simulink model "copter_simulink_control_trajectory_circle4"  (R2018b)
settings: Solver=ode45  StartTime=0.0  StopTime=200  FixedStep=.001  MaxStep=.05  MinStep=0.0001  RelTol=1e-3  EnableMultiTasking=on
libraries: simulink x10
settings Model: Creator=bengiami  LastModifiedBy=bengiami
settings SolverCC: MaxConsecutiveZCs=100  AutoInsertRateTranBlk=on
settings DataIOCC: LimitDataPoints=on  SaveFormat=Array  SaveOutput=off  SaveTime=off
settings OptimizationCC: DefaultParameterBehavior=Inlined  InlineInvariantSignals=on  StateBitsets=on  DataBitsets=on  ZeroExternalMemoryAtStartup=off  ZeroInternalMemoryAtStartup=off  NoFixptDivByZeroProtection=on  LifeSpan=1
settings DebuggingCC: AlgebraicLoopMsg=none  MaxConsecutiveZCsMsg=none  SolverPrmCheckMsg=warning  SFUnexpectedBacktrackingDiag=warning  SFNoUnconditionalDefaultTransitionDiag=warning  SFExecutionAtInitializationDiag=none
settings HardwareCC: ProdBitPerPointer=32  ProdBitPerSizeT=32  ProdBitPerPtrDiffT=32  ProdLargestAtomicFloat=None  ProdIntDivRoundTo=Floor  ProdWordSize=32  ProdHWDeviceType=Generic->Custom
settings ModelReferenceCC: PropagateSignalLabelsOutOfModel=off
settings SFSimCC: SimUseLocalCustomCode=off  MATLABDynamicMemAlloc=off
settings RTWCC: SystemTargetFile=ert.tlc  TLCOptions=-p0  GenCodeOnly=on  TemplateMakefile=ert_default_tmf  GenerateReport=on  RTWVerbose=off  RTWUseLocalCustomCode=off  IncludeHyperlinkInReport=on  LaunchReport=on
settings CodeAppCC: ForceParamTrailComments=on  IgnoreCustomStorageClasses=off  SimulinkDataObjDesc=on  CustomSymbolStrGlobalVar=rt$N$M  CustomSymbolStrType=$N$M  CustomSymbolStrFcn=$N$M$F  CustomSymbolStrMacro=$N$M  InsertBlockDesc=on  StateflowObjectComments=on
settings ERTTargetCC: CodeReplacementLibrary=ISO_C  MultiwordLength=2048  GenerateSampleERTMain=on  IncludeMdlTerminateFcn=off  SuppressErrorStatus=on  SupportAbsoluteTime=off  PurelyIntegerCode=on  SupportNonFinite=off  SupportComplex=off  InlinedParameterPlacement=NonHierarchical  RootIOFormat=Structure reference  ERTCustomFileTemplate=example_file_process.tlc  ConvertIfToSwitch=off  SuppressUnreachableDefaultCases=off
settings ConfigComp: CovMetricSettings=dw  CovHtmlReporting=on  CovSaveCumulativeToWorkspaceVar=on  CovSaveSingleToWorkspaceVar=on  CovExternalEMLEnable=off  CovSFcnEnable=off

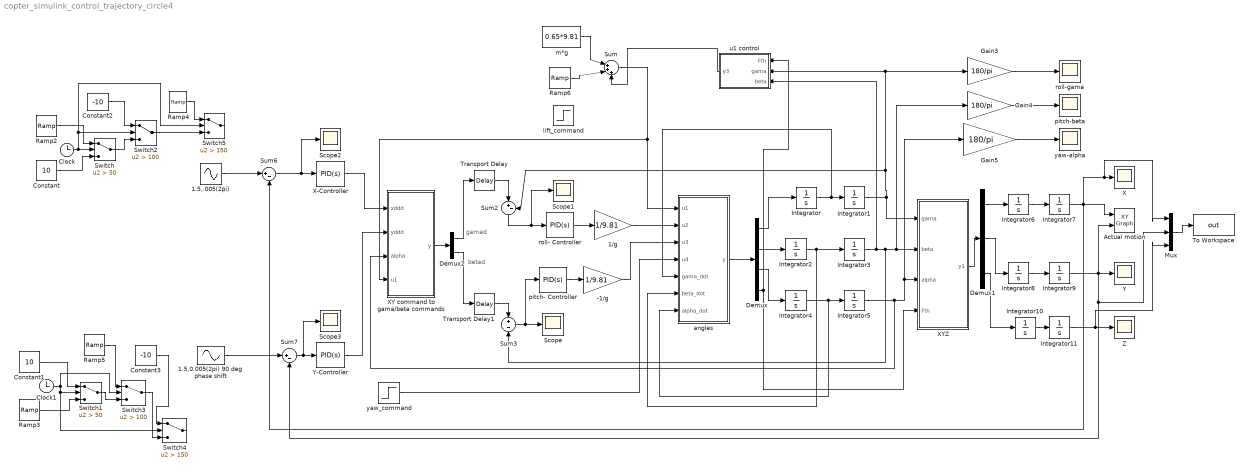
== system copter_simulink_control_trajectory_circle4 ==
  note: betad
  note: gamad
  -1/g : Gain  Gain=1/9.81
  1.5,.005(2pi) : Sin  Amplitude=10  Frequency=0.005*(2*pi)  SampleTime=0
  1.5,0.005(2pi) 90 deg phase shift : Sin  Amplitude=10  Frequency=0.005*(2*pi)  Phase=pi/2  SampleTime=0
  1/g : Gain  Gain=1/9.81
  Actual motion : simulink/Sinks/XY Graph  xmin=-25  xmax=25  ymin=-25  ymax=25  st=-1
  Clock : Clock
  Clock1 : Clock
  Constant : Constant  Value=10
  Constant1 : Constant  Value=10
  Constant2 : Constant  Value=-10
  Constant3 : Constant  Value=-10
  Demux : Demux
  Demux1 : Demux  Outputs=3
  Demux2 : Demux  Outputs=2
  Gain3 : Gain  Gain=180/pi
  Gain4 : Gain  Gain=180/pi
  Gain5 : Gain  Gain=180/pi
  Integrator{,1..8,10..11} (11 alike) : Integrator
  Integrator9 : Integrator  InitialCondition=10
  Mux : Mux  Inputs=3
  Ramp2 : simulink/Sources/Ramp  slope=-0.4  start=50  InitialOutput=10
  Ramp3 : simulink/Sources/Ramp  slope=0.4  start=0  InitialOutput=-10
  Ramp4 : simulink/Sources/Ramp  slope=0.4  start=150  InitialOutput=-10
  Ramp5 : simulink/Sources/Ramp  slope=-0.4  start=100  InitialOutput=10
  Ramp6 : simulink/Sources/Ramp  slope=-0.0000001  start=0  InitialOutput=0
  Scope{,1..3} (4 alike) : Scope
  Sum : Sum  Inputs=|+++
  Sum2 : Sum  Inputs=|+-
  Sum3 : Sum  Inputs=+-
  Sum6 : Sum  Inputs=|+-
  Sum7 : Sum  Inputs=|+-
  Switch : Switch  Criteria=u2 > Threshold  Threshold=50
  Switch1 : Switch  Criteria=u2 > Threshold  Threshold=50
  Switch2 : Switch  Criteria=u2 > Threshold  Threshold=100
  Switch3 : Switch  Criteria=u2 > Threshold  Threshold=100
  Switch4 : Switch  Criteria=u2 > Threshold  Threshold=150
  Switch5 : Switch  Criteria=u2 > Threshold  Threshold=150
  To Workspace : ToWorkspace  VariableName=out  SaveFormat=Timeseries  SampleTime=-1
  Transport Delay : TransportDelay  DelayTime=0.0001
  Transport Delay1 : TransportDelay  DelayTime=0.0001
  X : Scope
  X-Controller : simulink/Continuous/PID Controller  Controller=PID  Form=Parallel  TimeDomain=Continuous-time  SampleTime=1  IntegratorMethod=Forward Euler  FilterMethod=Forward Euler  ControllerParametersSource=internal  P=2  I=0.05  D=0.1  UseFilter=on  N=1000  TunerSelectOption=Transfer Function Based (PID Tuner App)  InitialConditionSource=internal  InitialConditionForIntegrator=0  InitialConditionForFilter=0  DifferentiatorICPrevScaledInput=0  ExternalReset=none  TrackingMode=off  Kt=1  LimitOutput=off  UpperSaturationLimit=inf  LowerSaturationLimit=-inf  LinearizeAsGain=on  AntiWindupMode=none  Kb=1  POutMin=[]  POutMax=[]  IOutMin=[]  IOutMax=[]  DOutMin=[]  DOutMax=[]  NOutMin=[]  NOutMax=[]  SumOutMin=[]  SumOutMax=[]  SaturationOutMin=[]  SaturationOutMax=[]  PParamMin=[]  PParamMax=[]  IParamMin=[]  IParamMax=[]  DParamMin=[]  DParamMax=[]  NParamMin=[]  NParamMax=[]  KbParamMin=[]  KbParamMax=[]  KtParamMin=[]  KtParamMax=[]  KbOutMin=[]  KbOutMax=[]  KtOutMin=[]  KtOutMax=[]  IntegratorOutMin=[]  IntegratorOutMax=[]  FilterOutMin=[]  FilterOutMax=[]  SumI1OutMin=[]  SumI1OutMax=[]  SumI2OutMin=[]  SumI2OutMax=[]  SumI3OutMin=[]  SumI3OutMax=[]  SumI4OutMin=[]  SumI4OutMax=[]  SumDOutMin=[]  SumDOutMax=[]  DifferentiatorOutMin=[]  DifferentiatorOutMax=[]  FilterDiffOutCoefMin=[]  FilterDiffOutCoefMax=[]  ReciprocalOutMin=[]  ReciprocalOutMax=[]  SumDenOutMin=[]  SumDenOutMax=[]  SumNumOutMin=[]  SumNumOutMax=[]  DivideOutMin=[]  DivideOutMax=[]  IntegratorContinuousStateAttributes=''  IntegratorStateMustResolveToSignalObject=off  IntegratorRTWStateStorageClass=Auto  FilterContinuousStateAttributes=''  FilterStateMustResolveToSignalObject=off  FilterRTWStateStorageClass=Auto  ParallelPVariant=InternalParameters  IdealPVariant=Disabled  IVariant=InternalParameters  DVariant=InternalParameters  IntegratorVariant=Continuous  SatVariant=Disabled  AWVariant=Passthrough  PCopyVariant=Disabled  TRVariant=Disabled  FdbkBlocksVariant=Forward  IdealPFdbkVariant=Disabled  SatFdbkVariant=Disabled  DerivativeFilterVariant=ContFilter  NVariant=InternalParameters  NCopyVariant=Disabled  FilterICVariant=InternalICsFilter  IntegratorICVariant=InternalICs  ExternalResetVariant=Disabled  TRSumVariant=Passthrough  SumFdbkVariant=Disabled  SumVariant=Sum_PID
  XY command to gama/beta commands : MATLAB Function  TreatAsAtomicUnit=on
  XYZ : MATLAB Function  TreatAsAtomicUnit=on
  Y : Scope
  Y-Controller : simulink/Continuous/PID Controller  Controller=PID  Form=Parallel  TimeDomain=Continuous-time  SampleTime=1  IntegratorMethod=Forward Euler  FilterMethod=Forward Euler  ControllerParametersSource=internal  P=2  I=0.05  D=0.13  UseFilter=on  N=1000  TunerSelectOption=Transfer Function Based (PID Tuner App)  InitialConditionSource=internal  InitialConditionForIntegrator=0  InitialConditionForFilter=0  DifferentiatorICPrevScaledInput=0  ExternalReset=none  TrackingMode=off  Kt=1  LimitOutput=off  UpperSaturationLimit=inf  LowerSaturationLimit=-inf  LinearizeAsGain=on  AntiWindupMode=none  Kb=1  POutMin=[]  POutMax=[]  IOutMin=[]  IOutMax=[]  DOutMin=[]  DOutMax=[]  NOutMin=[]  NOutMax=[]  SumOutMin=[]  SumOutMax=[]  SaturationOutMin=[]  SaturationOutMax=[]  PParamMin=[]  PParamMax=[]  IParamMin=[]  IParamMax=[]  DParamMin=[]  DParamMax=[]  NParamMin=[]  NParamMax=[]  KbParamMin=[]  KbParamMax=[]  KtParamMin=[]  KtParamMax=[]  KbOutMin=[]  KbOutMax=[]  KtOutMin=[]  KtOutMax=[]  IntegratorOutMin=[]  IntegratorOutMax=[]  FilterOutMin=[]  FilterOutMax=[]  SumI1OutMin=[]  SumI1OutMax=[]  SumI2OutMin=[]  SumI2OutMax=[]  SumI3OutMin=[]  SumI3OutMax=[]  SumI4OutMin=[]  SumI4OutMax=[]  SumDOutMin=[]  SumDOutMax=[]  DifferentiatorOutMin=[]  DifferentiatorOutMax=[]  FilterDiffOutCoefMin=[]  FilterDiffOutCoefMax=[]  ReciprocalOutMin=[]  ReciprocalOutMax=[]  SumDenOutMin=[]  SumDenOutMax=[]  SumNumOutMin=[]  SumNumOutMax=[]  DivideOutMin=[]  DivideOutMax=[]  IntegratorContinuousStateAttributes=''  IntegratorStateMustResolveToSignalObject=off  IntegratorRTWStateStorageClass=Auto  FilterContinuousStateAttributes=''  FilterStateMustResolveToSignalObject=off  FilterRTWStateStorageClass=Auto  ParallelPVariant=InternalParameters  IdealPVariant=Disabled  IVariant=InternalParameters  DVariant=InternalParameters  IntegratorVariant=Continuous  SatVariant=Disabled  AWVariant=Passthrough  PCopyVariant=Disabled  TRVariant=Disabled  FdbkBlocksVariant=Forward  IdealPFdbkVariant=Disabled  SatFdbkVariant=Disabled  DerivativeFilterVariant=ContFilter  NVariant=InternalParameters  NCopyVariant=Disabled  FilterICVariant=InternalICsFilter  IntegratorICVariant=InternalICs  ExternalResetVariant=Disabled  TRSumVariant=Passthrough  SumFdbkVariant=Disabled  SumVariant=Sum_PID
  Z : Scope
  angles : MATLAB Function  TreatAsAtomicUnit=on
  lift_command : Step  Time=0  After=0  SampleTime=0
  m*g : Constant  Value=0.65*9.81
  pitch- Controller : simulink/Continuous/PID Controller  Controller=PID  Form=Parallel  TimeDomain=Continuous-time  SampleTime=1  IntegratorMethod=Forward Euler  FilterMethod=Forward Euler  ControllerParametersSource=internal  P=4  I=0.05  D=0.1  UseFilter=on  N=1000  TunerSelectOption=Transfer Function Based (PID Tuner App)  InitialConditionSource=internal  InitialConditionForIntegrator=0  InitialConditionForFilter=0  DifferentiatorICPrevScaledInput=0  ExternalReset=none  TrackingMode=off  Kt=1  LimitOutput=off  UpperSaturationLimit=inf  LowerSaturationLimit=-inf  LinearizeAsGain=on  AntiWindupMode=none  Kb=1  POutMin=[]  POutMax=[]  IOutMin=[]  IOutMax=[]  DOutMin=[]  DOutMax=[]  NOutMin=[]  NOutMax=[]  SumOutMin=[]  SumOutMax=[]  SaturationOutMin=[]  SaturationOutMax=[]  PParamMin=[]  PParamMax=[]  IParamMin=[]  IParamMax=[]  DParamMin=[]  DParamMax=[]  NParamMin=[]  NParamMax=[]  KbParamMin=[]  KbParamMax=[]  KtParamMin=[]  KtParamMax=[]  KbOutMin=[]  KbOutMax=[]  KtOutMin=[]  KtOutMax=[]  IntegratorOutMin=[]  IntegratorOutMax=[]  FilterOutMin=[]  FilterOutMax=[]  SumI1OutMin=[]  SumI1OutMax=[]  SumI2OutMin=[]  SumI2OutMax=[]  SumI3OutMin=[]  SumI3OutMax=[]  SumI4OutMin=[]  SumI4OutMax=[]  SumDOutMin=[]  SumDOutMax=[]  DifferentiatorOutMin=[]  DifferentiatorOutMax=[]  FilterDiffOutCoefMin=[]  FilterDiffOutCoefMax=[]  ReciprocalOutMin=[]  ReciprocalOutMax=[]  SumDenOutMin=[]  SumDenOutMax=[]  SumNumOutMin=[]  SumNumOutMax=[]  DivideOutMin=[]  DivideOutMax=[]  IntegratorContinuousStateAttributes=''  IntegratorStateMustResolveToSignalObject=off  IntegratorRTWStateStorageClass=Auto  FilterContinuousStateAttributes=''  FilterStateMustResolveToSignalObject=off  FilterRTWStateStorageClass=Auto  ParallelPVariant=InternalParameters  IdealPVariant=Disabled  IVariant=InternalParameters  DVariant=InternalParameters  IntegratorVariant=Continuous  SatVariant=Disabled  AWVariant=Passthrough  PCopyVariant=Disabled  TRVariant=Disabled  FdbkBlocksVariant=Forward  IdealPFdbkVariant=Disabled  SatFdbkVariant=Disabled  DerivativeFilterVariant=ContFilter  NVariant=InternalParameters  NCopyVariant=Disabled  FilterICVariant=InternalICsFilter  IntegratorICVariant=InternalICs  ExternalResetVariant=Disabled  TRSumVariant=Passthrough  SumFdbkVariant=Disabled  SumVariant=Sum_PID
  pitch-beta : Scope
  roll- Controller : simulink/Continuous/PID Controller  Controller=PID  Form=Parallel  TimeDomain=Continuous-time  SampleTime=1  IntegratorMethod=Forward Euler  FilterMethod=Forward Euler  ControllerParametersSource=internal  P=4  I=0.05  D=0.1  UseFilter=on  N=1000  TunerSelectOption=Transfer Function Based (PID Tuner App)  InitialConditionSource=internal  InitialConditionForIntegrator=0  InitialConditionForFilter=0  DifferentiatorICPrevScaledInput=0  ExternalReset=none  TrackingMode=off  Kt=1  LimitOutput=off  UpperSaturationLimit=inf  LowerSaturationLimit=-inf  LinearizeAsGain=on  AntiWindupMode=none  Kb=1  POutMin=[]  POutMax=[]  IOutMin=[]  IOutMax=[]  DOutMin=[]  DOutMax=[]  NOutMin=[]  NOutMax=[]  SumOutMin=[]  SumOutMax=[]  SaturationOutMin=[]  SaturationOutMax=[]  PParamMin=[]  PParamMax=[]  IParamMin=[]  IParamMax=[]  DParamMin=[]  DParamMax=[]  NParamMin=[]  NParamMax=[]  KbParamMin=[]  KbParamMax=[]  KtParamMin=[]  KtParamMax=[]  KbOutMin=[]  KbOutMax=[]  KtOutMin=[]  KtOutMax=[]  IntegratorOutMin=[]  IntegratorOutMax=[]  FilterOutMin=[]  FilterOutMax=[]  SumI1OutMin=[]  SumI1OutMax=[]  SumI2OutMin=[]  SumI2OutMax=[]  SumI3OutMin=[]  SumI3OutMax=[]  SumI4OutMin=[]  SumI4OutMax=[]  SumDOutMin=[]  SumDOutMax=[]  DifferentiatorOutMin=[]  DifferentiatorOutMax=[]  FilterDiffOutCoefMin=[]  FilterDiffOutCoefMax=[]  ReciprocalOutMin=[]  ReciprocalOutMax=[]  SumDenOutMin=[]  SumDenOutMax=[]  SumNumOutMin=[]  SumNumOutMax=[]  DivideOutMin=[]  DivideOutMax=[]  IntegratorContinuousStateAttributes=''  IntegratorStateMustResolveToSignalObject=off  IntegratorRTWStateStorageClass=Auto  FilterContinuousStateAttributes=''  FilterStateMustResolveToSignalObject=off  FilterRTWStateStorageClass=Auto  ParallelPVariant=InternalParameters  IdealPVariant=Disabled  IVariant=InternalParameters  DVariant=InternalParameters  IntegratorVariant=Continuous  SatVariant=Disabled  AWVariant=Passthrough  PCopyVariant=Disabled  TRVariant=Disabled  FdbkBlocksVariant=Forward  IdealPFdbkVariant=Disabled  SatFdbkVariant=Disabled  DerivativeFilterVariant=ContFilter  NVariant=InternalParameters  NCopyVariant=Disabled  FilterICVariant=InternalICsFilter  IntegratorICVariant=InternalICs  ExternalResetVariant=Disabled  TRSumVariant=Passthrough  SumFdbkVariant=Disabled  SumVariant=Sum_PID
  roll-gama : Scope
  u1 control : MATLAB Function  TreatAsAtomicUnit=on
  yaw-alpha : Scope
  yaw_command : Step  Time=0.25  After=0  SampleTime=0
  wires:
  yaw_command/1 -> angles/4(u4)
  angles/1(y) -> Demux/1
  Demux/2 -> Integrator2/1
  Demux/3 -> Integrator4/1
  XYZ/1(y1) -> Demux1/1
  Demux/4 -> XYZ/4(Fth), u1 control/1(Fth)
  Gain3/1 -> roll-gama/1
  Gain4/1 -> pitch-beta/1
  Gain5/1 -> yaw-alpha/1
  m*g/1 -> Sum/1
  Integrator5/1 -> XY command to gama/beta commands/3(alpha), Gain5/1, XYZ/3(alpha)
  Demux/1 -> Integrator/1
  Integrator10/1 -> Integrator11/1
  Integrator8/1 -> Integrator9/1
  Demux1/1 -> Integrator6/1
  Demux1/2 -> Integrator8/1
  Demux1/3 -> Integrator10/1
  Integrator2/1 -> Integrator3/1, angles/6(beta_dot)
  Integrator1/1 -> Sum2/2, u1 control/2(gama), Gain3/1, XYZ/1(gama)
  Integrator3/1 -> u1 control/3(beta), Sum3/2, Gain4/1, XYZ/2(beta)
  Integrator4/1 -> Integrator5/1, angles/7(alpha_dot)
  Integrator11/1 -> Z/1, Mux/3
  Integrator/1 -> angles/5(gama_dot), Integrator1/1
  Integrator7/1 -> Sum6/2, Actual motion/1, Mux/1, X/1
  Integrator9/1 -> Mux/2, Sum7/2, Actual motion/2, Y/1
  Integrator6/1 -> Integrator7/1
  Sum2/1 -> Scope1/1, roll- Controller/1
  Sum7/1 -> Y-Controller/1, Scope3/1
  Sum6/1 -> X-Controller/1, Scope2/1
  roll- Controller/1 -> 1/g/1
  pitch- Controller/1 -> -1/g/1
  X-Controller/1 -> XY command to gama/beta commands/1(xddd)
  Y-Controller/1 -> XY command to gama/beta commands/2(yddd)
  XY command to gama/beta commands/1(y) -> Demux2/1
  Demux2/2 -> Transport Delay1/1
  Demux2/1 -> Transport Delay/1
  Transport Delay/1 -> Sum2/1
  1/g/1 -> angles/2(u2)
  -1/g/1 -> angles/3(u3)
  Transport Delay1/1 -> Sum3/1
  Sum3/1 -> Scope/1, pitch- Controller/1
  Clock/1 -> Switch/2, Switch5/2, Switch2/2
  Clock1/1 -> Switch4/2, Switch1/2, Switch3/2
  Ramp2/1 -> Switch/1
  Constant/1 -> Switch/3
  Ramp3/1 -> Switch1/3
  Constant1/1 -> Switch1/1
  Switch/1 -> Switch2/3
  Constant2/1 -> Switch2/1
  Switch2/1 -> Switch5/3
  Ramp4/1 -> Switch5/1
  Switch1/1 -> Switch3/3
  Switch3/1 -> Switch4/3
  Ramp5/1 -> Switch3/1
  Constant3/1 -> Switch4/1
  Mux/1 -> To Workspace/1
  Ramp6/1 -> Sum/2
  Sum/1 -> XY command to gama/beta commands/4(u1), angles/1(u1)
  u1 control/1(y3) -> Sum/3
  1.5,.005(2pi)/1 -> Sum6/1
  1.5,0.005(2pi) 90 deg phase shift/1 -> Sum7/1

== matlab function copter_simulink_control_trajectory_circle4/XYZ ==
  data: gama input; y1 output; beta input; alpha input; Fth input
function y1= fcn(gama,beta,alpha,Fth)

m=0.65;g=9.81;
 x_ddot= -(Fth/m)*((cos(gama)*sin(beta)*cos(alpha))+(sin(gama)*sin(alpha)));
  
 y_ddot= -(Fth/m)*((cos(gama).*sin(beta)*sin(alpha))-(sin(gama)*cos(alpha)));
 
 z_ddot= g-(Fth/m)*(cos(gama)*cos(beta));
   
y1 = [x_ddot y_ddot z_ddot];

== matlab function copter_simulink_control_trajectory_circle4/angles ==
  data: u1 input; y output; u2 input; u3 input; u4 input; gama_dot input; beta_dot input; alpha_dot input
function y = fcn(u1,u2,u3,u4,gama_dot,beta_dot,alpha_dot)
%#codegen
Ixx=7.5e-3; Iyy=7.5e-3; Izz=1.3e-2;L=0.23;
Jr=6e-5;km=7.5e-7;kf=3.13e-5;
    omega1_sq=((0.25/kf)*u1+(0.5/kf)*u3-(0.25/km)*u4);
    omega1=sqrt(abs(omega1_sq)); 
    omega2_sq=((0.25/kf)*u1-(0.5/kf)*u3-(0.25/km)*u4);
    omega2=sqrt(abs(omega2_sq)); 
    omega3_sq=((0.25/kf)*u1-(0.5/kf)*u2+(0.25/km)*u4);
    omega3=sqrt(abs(omega3_sq));
    omega4_sq=((0.25/kf)*u1+(0.5/kf)*u2+(0.25/km)*u4);
    omega4=sqrt(abs(omega4_sq));
    F1=kf*omega1_sq;F2=kf*omega2_sq;F3=kf*omega3_sq;F4=kf*omega4_sq; %force of each propeller
    Fth=(F1+F2+F3+F4);  %lift force
    Mb=[L*u2;L*u3;u4];  %moments for roll, pitch and yaw
     
  omegar=omega1+omega2-omega3-omega4;
  
   gama_ddot=(1/Ixx)*((-beta_dot*(Izz-Iyy)*alpha_dot)-(beta_dot*Jr*omegar)+Mb(1));
   beta_ddot=(1/Iyy)*((-alpha_dot*(Ixx-Izz)*gama_dot)+(gama_dot*Jr*omegar)+Mb(2));
   alpha_ddot=(1/Izz)*((-beta_dot*(Iyy-Ixx)*gama_dot)+Mb(3));
    
  
y = [gama_ddot beta_ddot alpha_ddot,Fth];

== matlab function copter_simulink_control_trajectory_circle4/u1 control ==
  data: Fth input; y3 output; gama input; beta input
function y3 = fcn(Fth,gama,beta)
%#codegen
du1=Fth*(1-cos(gama)*cos(beta));
y3 = du1;

== matlab function copter_simulink_control_trajectory_circle4/XY command to gama//beta commands ==
  data: xddd input; y output; yddd input; alpha input; u1 input
function y = fcn(xddd,yddd,alpha,u1)
m=0.65;
gamad=(m/u1)*(-(xddd*sin(alpha))+(yddd*cos(alpha)));
betad=(m/u1)*(-(xddd*cos(alpha))-(yddd*sin(alpha)));
y = [gamad betad];
